simulink model "serial_i2c_sensors_MPU9250"  (R2016b)
settings: Solver=FixedStepDiscrete  StartTime=0.0  StopTime=10.0  FixedStep=1e-3  RelTol=1e-3
libraries: mbed_lib x4, mbed_i2c_sensors x3
settings Model: Creator=Sven Lack  LastModifiedBy=oh
settings DataIOCC: LimitDataPoints=on  SaveFormat=Array
settings OptimizationCC: LifeSpan=1
settings DebuggingCC: SolverPrmCheckMsg=warning  SFUnexpectedBacktrackingDiag=warning  SFNoUnconditionalDefaultTransitionDiag=warning  SFExecutionAtInitializationDiag=none
settings HardwareCC: ProdBitPerPointer=32  ProdBitPerSizeT=32  ProdBitPerPtrDiffT=32  ProdLargestAtomicInteger=Long  ProdLargestAtomicFloat=Double  ProdIntDivRoundTo=Undefined  ProdWordSize=32  ProdHWDeviceType=ARM Compatible->ARM Cortex
settings ModelReferenceCC: PropagateSignalLabelsOutOfModel=off
settings RTWCC: SystemTargetFile=mbed.tlc  TemplateMakefile=mbed.tmf  Description=Mbed Target (Embedded Target)  TargetLang=C++
settings CodeAppCC: IgnoreCustomStorageClasses=off
settings STFCustomTargetCC: TargetLibSuffix=.a  GenerateSampleERTMain=on  CombineOutputUpdateFcns=on  ERTCustomFileBanners=on  SupportContinuousTime=off  SupportNonInlinedSFcns=off  RemoveResetFunc=on  MATLABClassNameForMDSCustomization=Simulink.SoftwareTarget.ERTCustomization  GRTInterface=off  SystemTargetFile=mbed.tlc
settings ERTTargetCC: GenerateSampleERTMain=on  ParMdlRefBuildCompliant=off  CompOptLevelCompliant=off  ConcurrentExecutionCompliant=off  ERTFirstTimeCompliant=off  ModelStepFunctionPrototypeControlCompliant=off  CPPClassGenCompliant=off  UseToolchainInfoCompliant=off  ERTCustomFileTemplate=mbed_file_process.tlc  ConvertIfToSwitch=off  SuppressUnreachableDefaultCases=off
settings ConfigComp: CovMetricSettings=dw  CovHtmlReporting=on  CovSaveCumulativeToWorkspaceVar=on  CovSaveSingleToWorkspaceVar=on  CovExternalEMLEnable=off  CovSFcnEnable=off

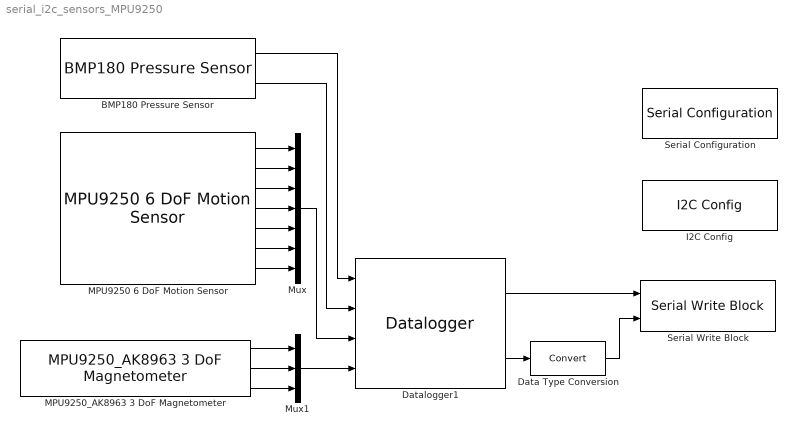
== system serial_i2c_sensors_MPU9250 ==
  BMP180 Pressure Sensor : mbed_i2c_sensors/BMP180 Pressure Sensor  i2cbus=1  SampleTime=0.1
  Data Type Conversion : DataTypeConversion
  Datalogger1 : mbed_lib/Utilities/Datalogger  TypeInputPorts={ 'int32' 1 'double' 1 'single' 7 'single' 3 }  TypeOfInputs={'1*int32' '1*double' '7*single' '3*single'}  BufferSize=1000  errEn=off  SampleTime=0.01
  I2C Config : mbed_lib/Serial/I2C/I2C Config  Priority=0  I2CPort=1  Freq=100000  SDAPortName=B  SDAPinNumber=9  SCLPortName=B  SCLPinNumber=8
  MPU9250 6 DoF Motion Sensor : mbed_i2c_sensors/MPU9250 6 DoF Motion Sensor  i2cbus=1  SubAddress=0xD0  SampleTime=0.01
  MPU9250_AK8963 3 DoF Magnetometer : mbed_i2c_sensors/MPU9250_AK8963 3 DoF Magnetometer  i2cbus=1  SubAddress=0x18  SampleTime=0.01
  Mux : Mux  Inputs=7
  Mux1 : Mux  Inputs=3
  Serial Configuration : mbed_lib/Serial/UART/Serial Configuration  SerialPort=1  TXPort=A  TXPin=2  RXPort=A  RXPin=3  BaudRate=9600
  Serial Write Block : mbed_lib/Serial/UART/Serial Write Block  SerialPort=1  numData=on  SampleTime=-1
  wires:
  Datalogger1/1 -> Serial Write Block/1
  BMP180 Pressure Sensor/2 -> Datalogger1/2
  BMP180 Pressure Sensor/1 -> Datalogger1/1
  Datalogger1/2 -> Data Type Conversion/1
  Data Type Conversion/1 -> Serial Write Block/2
  Mux/1 -> Datalogger1/3
  MPU9250 6 DoF Motion Sensor/2 -> Mux/2
  MPU9250 6 DoF Motion Sensor/1 -> Mux/1
  MPU9250 6 DoF Motion Sensor/7 -> Mux/7
  MPU9250 6 DoF Motion Sensor/4 -> Mux/4
  MPU9250 6 DoF Motion Sensor/6 -> Mux/6
  MPU9250 6 DoF Motion Sensor/3 -> Mux/3
  MPU9250 6 DoF Motion Sensor/5 -> Mux/5
  MPU9250_AK8963 3 DoF Magnetometer/1 -> Mux1/1
  MPU9250_AK8963 3 DoF Magnetometer/2 -> Mux1/2
  Mux1/1 -> Datalogger1/4
  MPU9250_AK8963 3 DoF Magnetometer/3 -> Mux1/3
